simulink model "SR26"  (R2025a)
settings: Solver=FixedStepDiscrete  StartTime=0.0  StopTime=100  FixedStep=0.01  RelTol=1e-3  EnableMultiTasking=on
PreLoadFcn:
  | try, model_open; catch, disp('Error occurred while executing model pre-load callback: model_open.m'); disp('Please assure that the MATLAB working directory is set to the model directory before opening.'); end
InitFcn:
  | try, model_open; catch, end
values from neighbouring files (symbols this model uses):
  dt = 10.0    [SR26.sldd]
undefined symbols (not defined in the file or in its folder): BMSInputProcessing, GCM, raptor_get_safe_string, raptor_xcp_function, RegenEnable, StateCAN, Subsystem, TCEnable
libraries: Utilities x263, Raptor_lib x137, simulink x7, IO x5, APPS_BSPC x4, TorqueCommand x3, Cooling x3, StateMachine x2, DriveSpeed x2, ATCC x2, BrakePressure x2, ThrottlePosition x2
(part 2 of 4)

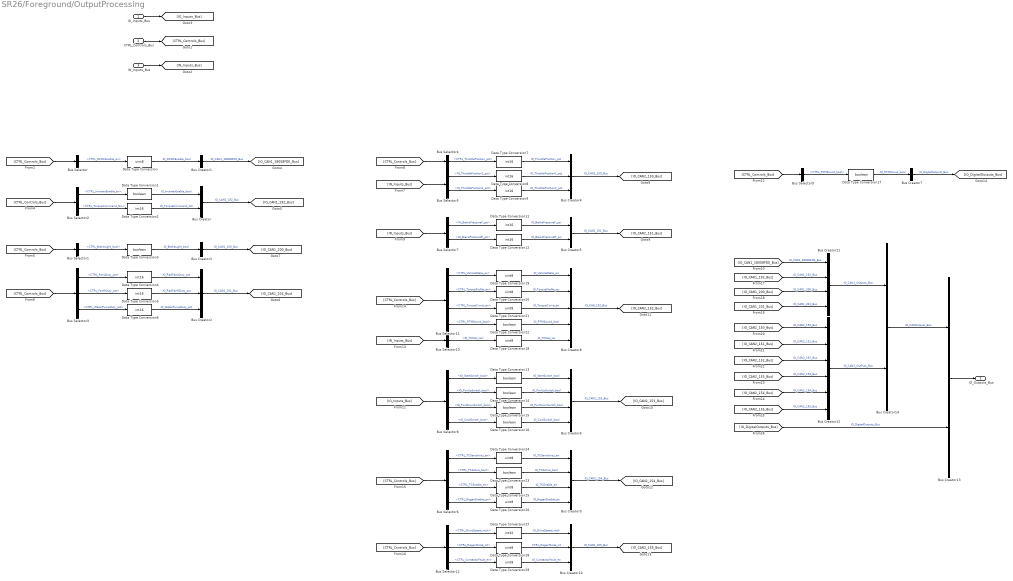
== system SR26/Foreground/OutputProcessing ==
  IO_Inputs_Bus : Inport
  CTRL_Controls_Bus : Inport  Port=2
  IN_Inputs_Bus : Inport  Port=3
  Bus Creator{,5,13..14} (4 alike) : BusCreator  Inputs=2
  Bus Creator1 : BusCreator  Inputs=1
  Bus Creator10 : BusCreator  Inputs=3
  Bus Creator11 : BusCreator  Inputs=4
  Bus Creator12 : BusCreator  Inputs=6
  Bus Creator2 : BusCreator  Inputs=3
  Bus Creator3 : BusCreator  Inputs=1
  Bus Creator4 : BusCreator  Inputs=3
  Bus Creator6 : BusCreator  Inputs=4
  Bus Creator7 : BusCreator  Inputs=1
  Bus Creator8 : BusCreator  Inputs=5
  Bus Creator9 : BusCreator  Inputs=4
  Bus Selector : BusSelector  OutputSignals=CTRL_DCDCEnable_en
  Bus Selector1 : BusSelector  OutputSignals=CTRL_BrakeLight_bool
  Bus Selector10 : BusSelector  OutputSignals=IN_TCDial_na
  Bus Selector11 : BusSelector  OutputSignals=CTRL_VehicleState_en,CTRL_TorqueProfile_en,CTRL_TorqueCurve_en,CTRL_RTMSound_bool
  Bus Selector12 : BusSelector  OutputSignals=CTRL_DriveSpeed_mph,CTRL_RegenMode_int,CTRL_ContactorFault_en
  Bus Selector2 : BusSelector  OutputSignals=CTRL_InverterEnable_en,CTRL_TorqueCommand_Nm
  Bus Selector3 : BusSelector  OutputSignals=CTRL_FanLDuty_pct,CTRL_FanRDuty_pct,CTRL_WaterPumpDuty_pct
  Bus Selector4 : BusSelector  OutputSignals=CTRL_ThrottlePosition_pct
  Bus Selector5 : BusSelector  OutputSignals=IN_ThrottlePosition_Bus.IN_ThrottlePosition1_pct,IN_ThrottlePosition_Bus.IN_ThrottlePosition2_pct
  Bus Selector6 : BusSelector  OutputSignals=CTRL_TCSensitivity_en,CTRL_TCActive_bool,CTRL_TCEnable_en,CTRL_RegenEnable_en
  Bus Selector7 : BusSelector  OutputSignals=IN_BrakePressure_Bus.IN_BrakePressureF_psi,IN_BrakePressure_Bus.IN_BrakePressureR_psi
  Bus Selector8 : BusSelector  OutputSignals=IO_DigitalInputs_Bus.IO_StartSwitch_bool,IO_DigitalInputs_Bus.IO_PwrUpSwitch_bool,IO_DigitalInputs_Bus.IO_PwrDownSwitch_bool,IO_DigitalInputs_Bus.IO_CoolSwitch_bool
  Bus Selector9 : BusSelector  OutputSignals=CTRL_RTMSound_bool
  Data Type Conversion{,18..21,24..26,28..29} (10 alike) : DataTypeConversion  OutDataTypeStr=uint8  SaturateOnIntegerOverflow=off  RndMeth=Floor
  Data Type Conversion{1,3,13..17,22..23} (9 alike) : DataTypeConversion  OutDataTypeStr=boolean  SaturateOnIntegerOverflow=off  RndMeth=Floor
  Data Type Conversion{2,4..9,11..12} (9 alike) : DataTypeConversion  OutDataTypeStr=int16  SaturateOnIntegerOverflow=off  RndMeth=Floor
  Data Type Conversion27 : DataTypeConversion  OutDataTypeStr=int32  SaturateOnIntegerOverflow=off  RndMeth=Floor
  IO_Outputs_Bus : Outport
  wires:
  IO_Inputs_Bus/1 -> [IO_Inputs_Bus]
  CTRL_Controls_Bus/1 -> [CTRL_Controls_Bus]
  IN_Inputs_Bus/1 -> [IN_Inputs_Bus]
  [CTRL_Controls_Bus] -> Bus Selector/1
  Bus Selector/1 -> Data Type Conversion/1  "<CTRL_DCDCEnable_en>"
  Bus Creator1/1 -> [IO_CAN1_18008FD0_Bus]  "IO_CAN1_18008FD0_Bus"
  [CTRL_Controls_Bus] -> Bus Selector2/1
  Bus Selector2/1 -> Data Type Conversion1/1  "<CTRL_InverterEnable_en>"
  Bus Selector2/2 -> Data Type Conversion2/1  "<CTRL_TorqueCommand_Nm>"
  Data Type Conversion2/1 -> Bus Creator/2  "IO_TorqueCommand_Nm"
  Data Type Conversion1/1 -> Bus Creator/1  "IO_InverterEnable_bool"
  Data Type Conversion/1 -> Bus Creator1/1  "IO_DCDCEnable_bool"
  Bus Creator/1 -> [IO_CAN1_192_Bus]  "IO_CAN1_192_Bus"
  [CTRL_Controls_Bus] -> Bus Selector1/1
  Bus Selector1/1 -> Data Type Conversion3/1  "<CTRL_BrakeLight_bool>"
  [CTRL_Controls_Bus] -> Bus Selector3/1
  Bus Selector3/1 -> Data Type Conversion4/1  "<CTRL_FanLDuty_pct>"
  Bus Selector3/2 -> Data Type Conversion5/1  "<CTRL_FanRDuty_pct>"
  Bus Selector3/3 -> Data Type Conversion6/1  "<CTRL_WaterPumpDuty_pct>"
  Data Type Conversion4/1 -> Bus Creator2/1  "IO_RadFanLDuty_pct"
  Data Type Conversion5/1 -> Bus Creator2/2  "IO_RadFanRDuty_pct"
  Data Type Conversion6/1 -> Bus Creator2/3  "IO_WaterPumpDuty_pct"
  Bus Creator2/1 -> [IO_CAN1_201_Bus]  "IO_CAN1_201_Bus"
  Data Type Conversion3/1 -> Bus Creator3/1  "IO_BrakeLight_bool"
  Bus Creator3/1 -> [IO_CAN1_200_Bus]  "IO_CAN1_200_Bus"
  [CTRL_Controls_Bus] -> Bus Selector4/1
  Bus Selector4/1 -> Data Type Conversion7/1  "<CTRL_ThrottlePosition_pct>"
  Data Type Conversion7/1 -> Bus Creator4/1  "IO_ThrottlePosition_pct"
  Bus Creator4/1 -> [IO_CAN2_150_Bus]  "IO_CAN1_150_Bus"
  [IN_Inputs_Bus] -> Bus Selector5/1
  Bus Selector5/1 -> Data Type Conversion8/1  "<IN_ThrottlePosition1_pct>"
  Bus Selector5/2 -> Data Type Conversion9/1  "<IN_ThrottlePosition2_pct>"
  Data Type Conversion8/1 -> Bus Creator4/2  "IO_ThrottlePosition1_pct"
  Data Type Conversion9/1 -> Bus Creator4/3  "IO_ThrottlePosition2_pct"
  Data Type Conversion12/1 -> Bus Creator5/2  "IO_BrakePressureR_psi"
  Data Type Conversion11/1 -> Bus Creator5/1  "IO_BrakePressureF_psi"
  [IN_Inputs_Bus] -> Bus Selector7/1
  Bus Creator5/1 -> [IO_CAN2_151_Bus]  "IO_CAN2_151_Bus"
  Bus Selector7/1 -> Data Type Conversion11/1  "<IN_BrakePressureF_psi>"
  Bus Selector7/2 -> Data Type Conversion12/1  "<IN_BrakePressureR_psi>"
  [IO_Inputs_Bus] -> Bus Selector8/1
  Bus Selector8/4 -> Data Type Conversion16/1  "<IO_CoolSwitch_bool>"
  Bus Selector8/3 -> Data Type Conversion15/1  "<IO_PwrDownSwitch_bool>"
  Bus Selector8/2 -> Data Type Conversion14/1  "<IO_PwrUpSwitch_bool>"
  Bus Selector8/1 -> Data Type Conversion13/1  "<IO_StartSwitch_bool>"
  Data Type Conversion13/1 -> Bus Creator6/1  "IO_StartSwitch_bool"
  Data Type Conversion14/1 -> Bus Creator6/2  "IO_PwrUpSwitch_bool"
  Data Type Conversion15/1 -> Bus Creator6/3  "IO_PwrDownSwitch_bool"
  Data Type Conversion16/1 -> Bus Creator6/4  "IO_CoolSwitch_bool"
  Bus Creator6/1 -> [IO_CAN2_153_Bus]  "IO_CAN2_153_Bus"
  [CTRL_Controls_Bus] -> Bus Selector9/1
  Bus Selector9/1 -> Data Type Conversion17/1  "<CTRL_RTMSound_bool>"
  Data Type Conversion17/1 -> Bus Creator7/1  "IO_RTMSound_bool"
  Bus Creator7/1 -> [IO_DigitalOutputs_Bus]  "IO_DigitalOutputs_Bus"
  Bus Creator8/1 -> [IO_CAN2_152_Bus]  "IO_CAN_152_Bus"
  Bus Selector10/1 -> Data Type Conversion18/1  "<IN_TCDial_na>"
  [IN_Inputs_Bus] -> Bus Selector10/1
  [CTRL_Controls_Bus] -> Bus Selector11/1
  Bus Selector11/1 -> Data Type Conversion19/1  "<CTRL_VehicleState_en>"
  Bus Selector11/2 -> Data Type Conversion20/1  "<CTRL_TorqueProfile_en>"
  Bus Selector11/3 -> Data Type Conversion21/1  "<CTRL_TorqueCurve_en>"
  Bus Selector11/4 -> Data Type Conversion22/1  "<CTRL_RTMSound_bool>"
  Data Type Conversion19/1 -> Bus Creator8/1  "IO_VehicleState_en"
  Data Type Conversion20/1 -> Bus Creator8/2  "IO_TorqueProfile_en"
  Data Type Conversion21/1 -> Bus Creator8/3  "IO_TorqueCurve_en"
  Data Type Conversion22/1 -> Bus Creator8/4  "IO_RTMSound_bool"
  Data Type Conversion18/1 -> Bus Creator8/5  "IO_TCDial_na"
  [CTRL_Controls_Bus] -> Bus Selector6/1
  Bus Selector6/1 -> Data Type Conversion24/1  "<CTRL_TCSensitivity_en>"
  Bus Selector6/2 -> Data Type Conversion23/1  "<CTRL_TCActive_bool>"
  Bus Selector6/3 -> Data Type Conversion25/1  "<CTRL_TCEnable_en>"
  Bus Selector6/4 -> Data Type Conversion26/1  "<CTRL_RegenEnable_en>"
  Data Type Conversion23/1 -> Bus Creator9/2  "IO_TCActive_bool"
  Data Type Conversion24/1 -> Bus Creator9/1  "IO_TCSensitivity_en"
  Data Type Conversion25/1 -> Bus Creator9/3  "IO_TCEnable_en"
  Data Type Conversion26/1 -> Bus Creator9/4  "IO_RegenEnable_en"
  Bus Creator9/1 -> [IO_CAN2_154_Bus]  "IO_CAN2_154_Bus"
  [CTRL_Controls_Bus] -> Bus Selector12/1
  Bus Selector12/1 -> Data Type Conversion27/1  "<CTRL_DriveSpeed_mph>"
  Bus Selector12/2 -> Data Type Conversion28/1  "<CTRL_RegenMode_int>"
  Bus Selector12/3 -> Data Type Conversion29/1  "<CTRL_ContactorFault_en>"
  Data Type Conversion29/1 -> Bus Creator10/3  "IO_ContactorFault_en"
  Data Type Conversion28/1 -> Bus Creator10/2  "CTRL_RegenMode_int"
  Data Type Conversion27/1 -> Bus Creator10/1  "IO_DriveSpeed_mph"
  Bus Creator10/1 -> [IO_CAN2_155_Bus]  "IO_CAN2_155_Bus"
  [IO_CAN1_18008FD0_Bus] -> Bus Creator11/1  "IO_CAN1_18008FD0_Bus"
  [IO_CAN1_192_Bus] -> Bus Creator11/2  "IO_CAN1_192_Bus"
  [IO_CAN1_200_Bus] -> Bus Creator11/3  "IO_CAN1_200_Bus"
  [IO_CAN1_201_Bus] -> Bus Creator11/4  "IO_CAN1_201_Bus"
  [IO_CAN2_150_Bus] -> Bus Creator12/1  "IO_CAN2_150_Bus"
  [IO_CAN2_151_Bus] -> Bus Creator12/2  "IO_CAN2_151_Bus"
  [IO_CAN2_152_Bus] -> Bus Creator12/3  "IO_CAN2_152_Bus"
  [IO_CAN2_153_Bus] -> Bus Creator12/4  "IO_CAN2_153_Bus"
  [IO_CAN2_154_Bus] -> Bus Creator12/5  "IO_CAN2_154_Bus"
  [IO_CAN2_155_Bus] -> Bus Creator12/6  "IO_CAN2_155_Bus"
  [IO_DigitalOutputs_Bus] -> Bus Creator13/2  "IO_DigitalOutputs_Bus"
  Bus Creator13/1 -> IO_Outputs_Bus/1
  Bus Creator11/1 -> Bus Creator14/1  "IO_CAN1_Outputs_Bus"
  Bus Creator12/1 -> Bus Creator14/2  "IO_CAN2_OutPuts_Bus"
  Bus Creator14/1 -> Bus Creator13/1  "IO_CANOutputs_Bus"

== system SR26/Power Up_Down/Background ==
  note: Notes :
      | - Calling the shutdown task stops the foreground tasks. However, background tasks continue, so the reading of key switch must be in this subsystem to allow the module
      | to resume operation (by calling the startup task) if keyswitch is turned back on before the module actually turns off.
      | - The Startup Event is automatically called when the module is powered on after being completely off. The FgndTasksStopped data store prevents the Startup Event from being called twice in this scenario.
  f : TriggerPort  TriggerType=function-call  VariantControl=Variant  ZeroCross=off
  Debounce : Subsystem
  Logical Operator1 : Logic  Operator=OR  OutDataTypeStr=boolean
  Logical Operator2 : Logic  Operator=OR  Inputs=3  OutDataTypeStr=boolean
  Raise Shutdown Event : Subsystem  TreatAsAtomicUnit=on
  Raise Startup Event : Subsystem  TreatAsAtomicUnit=on
  Store EEPROM : Subsystem  TreatAsAtomicUnit=on
  Unit Delay : UnitDelay  SampleTime=-1  HasFrameUpgradeWarning=on
  Unit Delay1 : UnitDelay  SampleTime=-1  HasFrameUpgradeWarning=on
  raptor_data_def : Raptor_lib/Data Storage/raptor_data_def  dataName='KeySw_Bgnd'  initValue=0  dataType=boolean  storage=Volatile (RAM)  calVisible=on  calType=Measurement  calDispType=Number  calEnum={'False', 'True'}  calGain=1.0  calOffset=0  calMin=-Inf  calMax=Inf  calFormat='-1'  calUnit='Bool'  calHelp='Key switch reading from background task'  calAccess=1  calFunction=group  calDispHeaders=off  calColHeaders={'Col1' 'Col2' 'Col3'}  calRowHeaders={'Row1' 'Row2' 'Row3'}
      settings: SourceProductName=Raptor
  raptor_data_def1 : Raptor_lib/Data Storage/raptor_data_def  dataName='KeepModuleOn'  initValue=0  dataType=boolean  storage=Volatile (RAM)  calVisible=on  calType=Measurement  calDispType=Number  calEnum={'False', 'True'}  calGain=1.0  calOffset=0  calMin=-Inf  calMax=Inf  calFormat='-1'  calUnit='Bool'  calHelp='Boolean indicating module to be kept on'  calAccess=1  calFunction=group  calDispHeaders=off  calColHeaders={'Col1' 'Col2' 'Col3'}  calRowHeaders={'Row1' 'Row2' 'Row3'}
      settings: SourceProductName=Raptor
  raptor_data_read : Raptor_lib/Data Storage/raptor_data_read  dataName='FgndTasksStopped'  dataShape=Scalar  idxSource=Input  idxRow=1  idxCol=1
      settings: SourceProductName=Raptor
  raptor_data_read1 : Raptor_lib/Data Storage/raptor_data_read  dataName='KeepModuleOn'  dataShape=Scalar  idxSource=Input  idxRow=1  idxCol=1
      settings: SourceProductName=Raptor
  raptor_data_write : Raptor_lib/Data Storage/raptor_data_write  dataName='KeySw_Bgnd'  dataShape=Scalar  idxSource=Input Port  idxRow=1  idxCol=1
      settings: SourceProductName=Raptor
  raptor_digital_in : Raptor_lib/Input & Output/raptor_digital_in  resourceValues=WAKE_INPUT1|INPUT33|INPUT34|INPUT35|INPUT36|INPUT37|INPUT38|INPUT39|INPUT40|(None)  resource=WAKE_INPUT1  pullUDValues=2.9k PD  pullUD=2.9k PD  upperThres=1.980  lowerThres=1.320
      settings: SourceProductName=Raptor
  raptor_digital_out : Raptor_lib/Input & Output/raptor_digital_out  resourceValues=OUTPUT9|OUTPUT21|OUTPUT22|OUTPUT23|OUTPUT24|(None)|OUTPUT1|OUTPUT2|OUTPUT3|OUTPUT4|OUTPUT5|OUTPUT6|OUTPUT7|OUTPUT8|OUTPUT10|OUTPUT11|OUTPUT25|OUTPUT26|OUTPUT27|OUTPUT28|OUTPUT29|OUTPUT30|OUTPUT31|OUTPUT32|OUTPUT33|OUTPUT34|OUTPUT35|OUTPUT36|OUTPUT37|OUTPUT38|OUTPUT39|OUTPUT40|OUTPUT41|OUTPUT42|OUTPUT43|OUTPUT44|OUTPUT45|OUTPUT46|OUTPUT47|OUTPUT48|POWER_HOLD  resource=POWER_HOLD  driverTypeValues=(None)  driverType=(None)
      settings: SourceProductName=Raptor
  raptor_sfun_nv_status : Raptor_lib/Data Storage/raptor_sfun_nv_status  showStatus=Store In Progess
      settings: SourceProductName=Raptor
  wires:
  raptor_data_read/1 -> Raise Startup Event/Enable
  raptor_digital_in/1 -> Debounce/1(In)
  Logical Operator2/1 -> raptor_digital_out/1
  Unit Delay/1 -> Store EEPROM/Trigger, Unit Delay1/1
  Logical Operator1/1 -> Logical Operator2/2, Raise Startup Event/Trigger, Raise Shutdown Event/Trigger, Unit Delay/1
  Unit Delay1/1 -> Logical Operator2/3
  raptor_sfun_nv_status/1 -> Logical Operator2/1
  raptor_data_read1/1 -> Logical Operator1/2
  Debounce/1(Out) -> raptor_data_write/1, Logical Operator1/1

== system SR26/Foreground/Controls Algorithm/APPS_BSPC ==
  IN_Inputs_Bus : Inport
  function : TriggerPort  TriggerType=function-call  VariantControl=(inherit)
  APPS : APPS_BSPC/APPS  SystemSampleTime=-1  VariantActivationTime=update diagram  EmptyChoice=off  PassThrough=off  PassThroughVariantControl=(default)  EmptyChoiceVariantControl=(default)  AllowFlexibleInterface=on  Latency=0  AutoFrameSizeCalculation=off
  BSPC : APPS_BSPC/BSPC  SystemSampleTime=-1  VariantActivationTime=update diagram  EmptyChoice=off  PassThrough=off  PassThroughVariantControl=(default)  EmptyChoiceVariantControl=(default)  AllowFlexibleInterface=on  Latency=0  AutoFrameSizeCalculation=off
  BSPCReset : APPS_BSPC/BSPCReset  SystemSampleTime=-1  VariantActivationTime=update diagram  EmptyChoice=off  PassThrough=off  PassThroughVariantControl=(default)  EmptyChoiceVariantControl=(default)  AllowFlexibleInterface=on  Latency=0  AutoFrameSizeCalculation=off
  Bus Selector : BusSelector  OutputSignals=IN_ThrottlePosition_Bus.IN_ThrottlePosition1_pct,IN_ThrottlePosition_Bus.IN_ThrottlePosition2_pct,IN_BrakePressure_Bus.IN_BrakePressureF_psi,IN_BrakePressure_Bus.IN_BrakePressureR_psi
  ThrottleSignal : APPS_BSPC/ThrottleSignal  SystemSampleTime=-1  VariantActivationTime=update diagram  EmptyChoice=off  PassThrough=off  PassThroughVariantControl=(default)  EmptyChoiceVariantControl=(default)  AllowFlexibleInterface=on  Latency=0  AutoFrameSizeCalculation=off
  CTRL_ThrottlePosition_pct : Outport
  wires:
  IN_Inputs_Bus/1 -> Bus Selector/1
  ThrottleSignal/1 -> CTRL_ThrottlePosition_pct/1
  Bus Selector/1 -> BSPC/1, BSPCReset/1, ThrottleSignal/1, APPS/1  "<IN_ThrottlePosition1_pct>"
  Bus Selector/2 -> BSPC/2, BSPCReset/2, ThrottleSignal/2, APPS/2  "<IN_ThrottlePosition2_pct>"
  Bus Selector/3 -> BSPC/3  "<IN_BrakePressureF_psi>"
  Bus Selector/4 -> BSPC/4  "<IN_BrakePressureR_psi>"

== system SR26/Foreground/Controls Algorithm/BrakeLight ==
  IN_Inputs_Bus : Inport
  function : TriggerPort  TriggerType=function-call  VariantControl=(inherit)
  BrakeLight : Brakes/BrakeLight  SystemSampleTime=-1  VariantActivationTime=update diagram  EmptyChoice=off  PassThrough=off  PassThroughVariantControl=(default)  EmptyChoiceVariantControl=(default)  AllowFlexibleInterface=on  Latency=0  AutoFrameSizeCalculation=off
  Bus Selector : BusSelector  OutputSignals=IN_BrakePressure_Bus.IN_BrakePressureF_psi,IN_BrakePressure_Bus.IN_BrakePressureR_psi
  CTRL_BrakeLight_bool : Outport
  wires:
  IN_Inputs_Bus/1 -> Bus Selector/1
  Bus Selector/1 -> BrakeLight/1  "<IN_BrakePressureF_psi>"
  Bus Selector/2 -> BrakeLight/2  "<IN_BrakePressureR_psi>"
  BrakeLight/1 -> CTRL_BrakeLight_bool/1

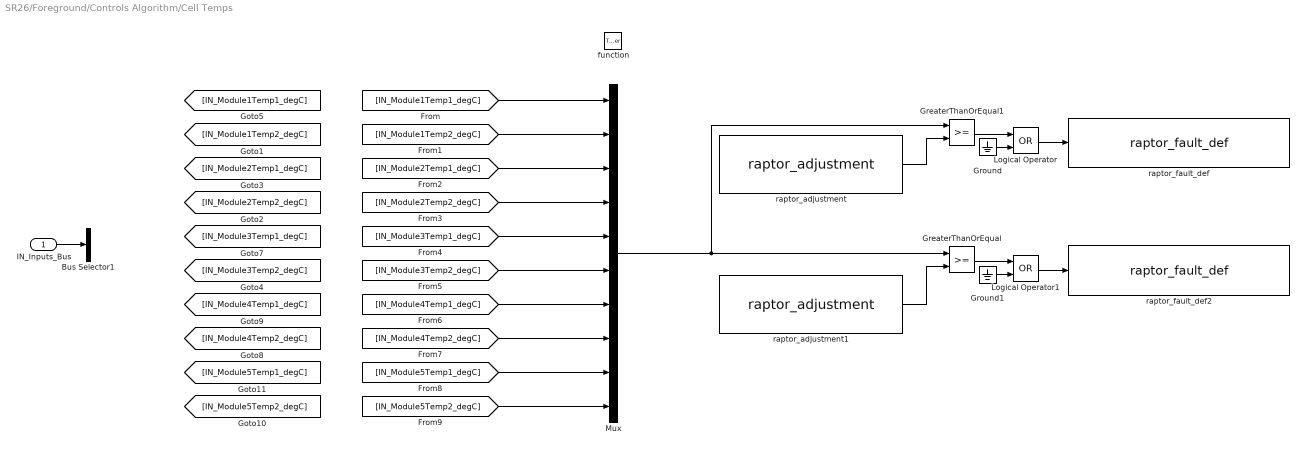
== system SR26/Foreground/Controls Algorithm/Cell Temps ==
  IN_Inputs_Bus : Inport
  function : TriggerPort  TriggerType=function-call  VariantControl=(inherit)
  Bus Selector1 : BusSelector  OutputSignals=IO_DigitalInputs_Bus.IO_CoolSwitch_bool
  GreaterThanOrEqual : RelationalOperator  OutDataTypeStr=boolean  RndMeth=Simplest  InputSameDT=off
  GreaterThanOrEqual1 : RelationalOperator  OutDataTypeStr=boolean  RndMeth=Simplest  InputSameDT=off
  Ground : Ground
  Ground1 : Ground
  Logical Operator : Logic  Operator=OR  AllPortsSameDT=off  OutDataTypeStr=boolean
  Logical Operator1 : Logic  Operator=OR  AllPortsSameDT=off  OutDataTypeStr=boolean
  Mux : Mux  Inputs=10
  raptor_adjustment : Raptor_lib/Data Storage/raptor_adjustment  paramName='CTRL_ModuleUnderThresh_degC'  nameSource=Parameter  initValue=-10  dataType=double  storage=Calibration  calDispType=Number  calEnum={'False', 'True'}  calGain=1.0  calOffset=0.0  calMax=inf  calMin=-inf  calFormat='-1'  calUnit=''  calHelp=''  calAccess=1  calFunction=raptor_xcp_function(gcb)  calDispHeaders=off  calColHeaders={'Col1' 'Col2' 'Col3'}  calRowHeaders={'Row1' 'Row2' 'Row3'}
      settings: SourceProductName=Raptor
  raptor_adjustment1 : Raptor_lib/Data Storage/raptor_adjustment  paramName='CTRL_ModuleOverTempThresh_degC'  nameSource=Parameter  initValue=55  dataType=double  storage=Calibration  calDispType=Number  calEnum={'False', 'True'}  calGain=1.0  calOffset=0.0  calMax=inf  calMin=-inf  calFormat='-1'  calUnit=''  calHelp=''  calAccess=1  calFunction=raptor_xcp_function(gcb)  calDispHeaders=off  calColHeaders={'Col1' 'Col2' 'Col3'}  calRowHeaders={'Row1' 'Row2' 'Row3'}
      settings: SourceProductName=Raptor
  raptor_fault_def : Raptor_lib/Faults/raptor_fault_def  faultName='CTRL_ModuleUnderTempFault'  persist=off  sticky=off  emisRelated=off  permanent=off  singleTrip=off  clearMethod=Standard  xLimit=25  yLimit=50  calEnable=on  addDisable=off  calAccess=1  calFunction='System | FaultManager'
      settings: SourceProductName=Raptor
  raptor_fault_def2 : Raptor_lib/Faults/raptor_fault_def  faultName='CTRL_ModuleOverTempTempFault'  persist=off  sticky=off  emisRelated=off  permanent=off  singleTrip=off  clearMethod=Standard  xLimit=25  yLimit=50  calEnable=on  addDisable=off  calAccess=1  calFunction='System | FaultManager'
      settings: SourceProductName=Raptor
  wires:
  IN_Inputs_Bus/1 -> Bus Selector1/1
  [IN_Module1Temp1_degC] -> Mux/1
  [IN_Module1Temp2_degC] -> Mux/2
  [IN_Module2Temp1_degC] -> Mux/3
  [IN_Module2Temp2_degC] -> Mux/4
  [IN_Module3Temp1_degC] -> Mux/5
  [IN_Module3Temp2_degC] -> Mux/6
  [IN_Module4Temp1_degC] -> Mux/7
  [IN_Module4Temp2_degC] -> Mux/8
  [IN_Module5Temp1_degC] -> Mux/9
  [IN_Module5Temp2_degC] -> Mux/10
  Mux/1 -> GreaterThanOrEqual1/1, GreaterThanOrEqual/1
  raptor_adjustment/1 -> GreaterThanOrEqual1/2
  raptor_adjustment1/1 -> GreaterThanOrEqual/2
  GreaterThanOrEqual1/1 -> Logical Operator/1
  Ground/1 -> Logical Operator/2
  Ground1/1 -> Logical Operator1/2
  GreaterThanOrEqual/1 -> Logical Operator1/1
  Logical Operator/1 -> raptor_fault_def/1
  Logical Operator1/1 -> raptor_fault_def2/1

== system SR26/Foreground/Controls Algorithm/ClearAllFaults ==
  function : TriggerPort  TriggerType=function-call  VariantControl=(inherit)
  raptor_fault_clear : Raptor_lib/Faults/raptor_fault_clear  faultSource=All  faultName='myFault'
      settings: SourceProductName=Raptor

== system SR26/Foreground/Controls Algorithm/RTMSound ==
  CTRL_VehicleState_en : Inport
  function : TriggerPort  TriggerType=function-call  VariantControl=(inherit)
  RTMSound : StateMachine/RTMSound  SystemSampleTime=-1  VariantActivationTime=update diagram  EmptyChoice=off  PassThrough=off  PassThroughVariantControl=(default)  EmptyChoiceVariantControl=(default)  AllowFlexibleInterface=on  Latency=0  AutoFrameSizeCalculation=off
  CTRL_RTMSound_bool : Outport
  wires:
  RTMSound/1 -> CTRL_RTMSound_bool/1
  CTRL_VehicleState_en/1 -> RTMSound/1

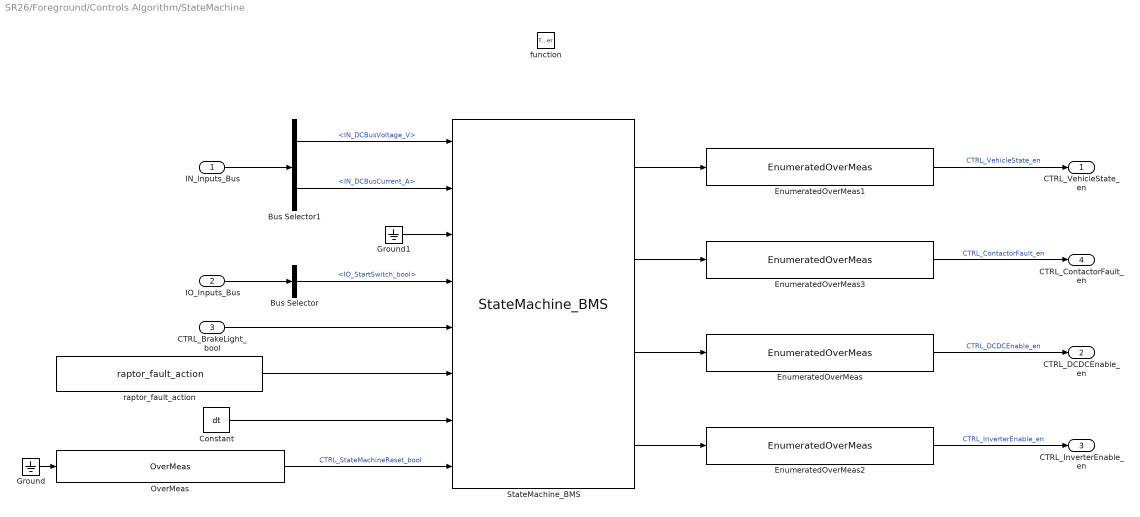
== system SR26/Foreground/Controls Algorithm/StateMachine ==
  IN_Inputs_Bus : Inport
  IO_Inputs_Bus : Inport  Port=2
  CTRL_BrakeLight_bool : Inport  Port=3
  function : TriggerPort  TriggerType=function-call  VariantControl=(inherit)
  Bus Selector : BusSelector  OutputSignals=IO_DigitalInputs_Bus.IO_StartSwitch_bool
  Bus Selector1 : BusSelector  OutputSignals=IN_CAN1_PM100DX_Bus.IN_DCBusVoltage_V,IN_CAN1_PM100DX_Bus.IN_DCBusCurrent_A
  Constant : Constant  Value=dt  OutDataTypeStr=uint32
  EnumeratedOverMeas : Utilities/EnumeratedOverMeas  sigName='CTRL_DCDCEnable_en'  enumName='DCDCEnable'
  EnumeratedOverMeas1 : Utilities/EnumeratedOverMeas  sigName='CTRL_VehicleState_en'  enumName='VehicleState'
  EnumeratedOverMeas2 : Utilities/EnumeratedOverMeas  sigName='CTRL_InverterEnable_en'  enumName='InverterEnable'
  EnumeratedOverMeas3 : Utilities/EnumeratedOverMeas  sigName='CTRL_ContactorFault_en'  enumName='ContactorFault'
  Ground : Ground
  Ground1 : Ground
  OverMeas : Utilities/OverMeas  sigName='CTRL_StateMachineReset_bool'  minimum=0  maximum=1
  StateMachine_BMS : StateMachine/StateMachine_BMS  SystemSampleTime=-1  VariantActivationTime=update diagram  EmptyChoice=off  PassThrough=off  PassThroughVariantControl=(default)  EmptyChoiceVariantControl=(default)  AllowFlexibleInterface=on  Latency=0  AutoFrameSizeCalculation=off
  raptor_fault_action : Raptor_lib/Faults/raptor_fault_action  actionName='myFaultAction'  calVisible=off  calAccess=1  calFunction='System | FaultManager | FaultAction'
      settings: SourceProductName=Raptor
  CTRL_VehicleState_en : Outport
  CTRL_DCDCEnable_en : Outport  Port=2
  CTRL_InverterEnable_en : Outport  Port=3
  CTRL_ContactorFault_en : Outport  Port=4
  wires:
  IO_Inputs_Bus/1 -> Bus Selector/1
  Bus Selector/1 -> StateMachine_BMS/4  "<IO_StartSwitch_bool>"
  IN_Inputs_Bus/1 -> Bus Selector1/1
  Bus Selector1/1 -> StateMachine_BMS/1  "<IN_DCBusVoltage_V>"
  Ground/1 -> OverMeas/1
  CTRL_BrakeLight_bool/1 -> StateMachine_BMS/5
  raptor_fault_action/1 -> StateMachine_BMS/6
  Constant/1 -> StateMachine_BMS/7
  OverMeas/1 -> StateMachine_BMS/8  "CTRL_StateMachineReset_bool"
  StateMachine_BMS/3 -> EnumeratedOverMeas/1
  StateMachine_BMS/1 -> EnumeratedOverMeas1/1
  StateMachine_BMS/4 -> EnumeratedOverMeas2/1
  EnumeratedOverMeas/1 -> CTRL_DCDCEnable_en/1  "CTRL_DCDCEnable_en"
  EnumeratedOverMeas2/1 -> CTRL_InverterEnable_en/1  "CTRL_InverterEnable_en"
  EnumeratedOverMeas1/1 -> CTRL_VehicleState_en/1  "CTRL_VehicleState_en"
  StateMachine_BMS/2 -> EnumeratedOverMeas3/1
  EnumeratedOverMeas3/1 -> CTRL_ContactorFault_en/1  "CTRL_ContactorFault_en"
  Ground1/1 -> StateMachine_BMS/3
  Bus Selector1/2 -> StateMachine_BMS/2  "<IN_DCBusCurrent_A>"

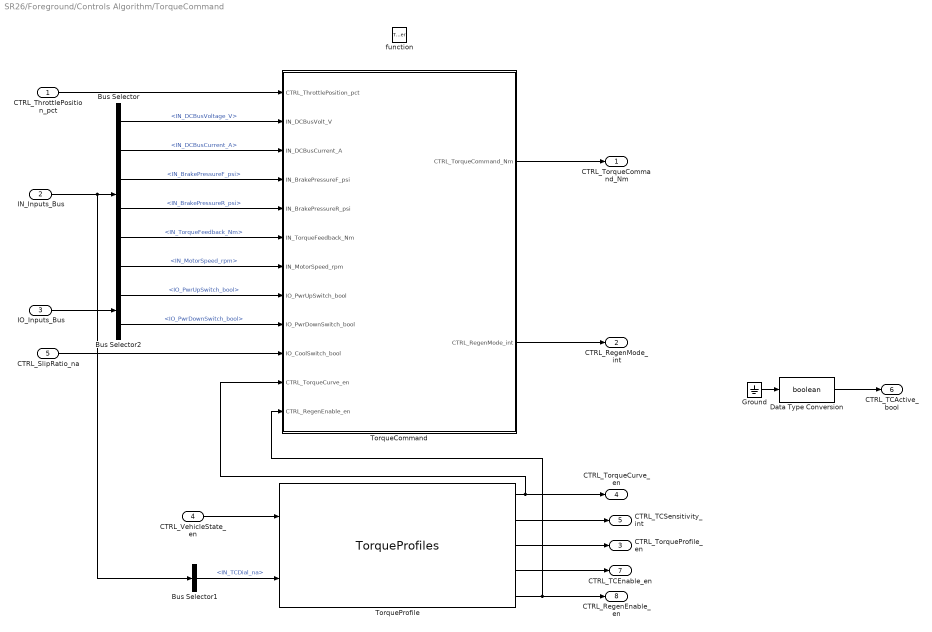
== system SR26/Foreground/Controls Algorithm/TorqueCommand ==
  CTRL_ThrottlePosition_pct : Inport
  IN_Inputs_Bus : Inport  Port=2
  IO_Inputs_Bus : Inport  Port=3
  CTRL_VehicleState_en : Inport  Port=4
  CTRL_SlipRatio_na : Inport  Port=5
  function : TriggerPort  TriggerType=function-call  VariantControl=(inherit)
  Bus Selector : BusSelector  OutputSignals=IN_CAN1_PM100DX_Bus.IN_DCBusVoltage_V,IN_CAN1_PM100DX_Bus.IN_DCBusCurrent_A,IN_BrakePressure_Bus.IN_BrakePressureF_psi,IN_BrakePressure_Bus.IN_BrakePressureR_psi,IN_CAN1_PM100DX_Bus.IN_TorqueFeedback_Nm,IN_CAN1_PM100DX_Bus.IN_MotorSpeed_rpm
  Bus Selector1 : BusSelector  OutputSignals=IN_TCDial_na
  Bus Selector2 : BusSelector  OutputSignals=IO_DigitalInputs_Bus.IO_PwrUpSwitch_bool,IO_DigitalInputs_Bus.IO_PwrDownSwitch_bool
  Data Type Conversion : DataTypeConversion  OutDataTypeStr=boolean  SaturateOnIntegerOverflow=off  RndMeth=Floor
  Ground : Ground
  TorqueCommand : Subsystem  AncestorBlock=TorqueCommand/TorqueCommand
  TorqueProfile : TorqueCommand/TorqueProfiles  SystemSampleTime=-1  VariantActivationTime=update diagram  EmptyChoice=off  PassThrough=off  PassThroughVariantControl=(default)  EmptyChoiceVariantControl=(default)  AllowFlexibleInterface=on  Latency=0  AutoFrameSizeCalculation=off
  CTRL_TorqueCommand_Nm : Outport  VectorParamsAs1DForOutWhenUnconnected=off
  CTRL_RegenMode_int : Outport  Port=2  VectorParamsAs1DForOutWhenUnconnected=off
  CTRL_TorqueProfile_en : Outport  Port=3  VectorParamsAs1DForOutWhenUnconnected=off
  CTRL_TorqueCurve_en : Outport  Port=4  VectorParamsAs1DForOutWhenUnconnected=off
  CTRL_TCSensitivity_int : Outport  Port=5  VectorParamsAs1DForOutWhenUnconnected=off
  CTRL_TCActive_bool : Outport  Port=6  VectorParamsAs1DForOutWhenUnconnected=off
  CTRL_TCEnable_en : Outport  Port=7  VectorParamsAs1DForOutWhenUnconnected=off
  CTRL_RegenEnable_en : Outport  Port=8  VectorParamsAs1DForOutWhenUnconnected=off
  wires:
  CTRL_ThrottlePosition_pct/1 -> TorqueCommand/1(CTRL_ThrottlePosition_pct)
  TorqueCommand/1(CTRL_TorqueCommand_Nm) -> CTRL_TorqueCommand_Nm/1
  IN_Inputs_Bus/1 -> Bus Selector1/1, Bus Selector/1
  TorqueProfile/1 -> TorqueCommand/11(CTRL_TorqueCurve_en), CTRL_TorqueCurve_en/1
  IO_Inputs_Bus/1 -> Bus Selector2/1
  Bus Selector1/1 -> TorqueProfile/2  "<IN_TCDial_na>"
  TorqueProfile/2 -> CTRL_TCSensitivity_int/1
  TorqueProfile/3 -> CTRL_TorqueProfile_en/1
  CTRL_VehicleState_en/1 -> TorqueProfile/1
  Bus Selector2/1 -> TorqueCommand/8(IO_PwrUpSwitch_bool)  "<IO_PwrUpSwitch_bool>"
  Bus Selector2/2 -> TorqueCommand/9(IO_PwrDownSwitch_bool)  "<IO_PwrDownSwitch_bool>"
  Bus Selector/3 -> TorqueCommand/4(IN_BrakePressureF_psi)  "<IN_BrakePressureF_psi>"
  Bus Selector/4 -> TorqueCommand/5(IN_BrakePressureR_psi)  "<IN_BrakePressureR_psi>"
  Bus Selector/5 -> TorqueCommand/6(IN_TorqueFeedback_Nm)  "<IN_TorqueFeedback_Nm>"
  Bus Selector/1 -> TorqueCommand/2(IN_DCBusVolt_V)  "<IN_DCBusVoltage_V>"
  Bus Selector/2 -> TorqueCommand/3(IN_DCBusCurrent_A)  "<IN_DCBusCurrent_A>"
  TorqueProfile/4 -> CTRL_TCEnable_en/1
  TorqueProfile/5 -> TorqueCommand/12(CTRL_RegenEnable_en), CTRL_RegenEnable_en/1
  Ground/1 -> Data Type Conversion/1
  Data Type Conversion/1 -> CTRL_TCActive_bool/1
  CTRL_SlipRatio_na/1 -> TorqueCommand/10(IO_CoolSwitch_bool)
  TorqueCommand/2(CTRL_RegenMode_int) -> CTRL_RegenMode_int/1
  Bus Selector/6 -> TorqueCommand/7(IN_MotorSpeed_rpm)  "<IN_MotorSpeed_rpm>"

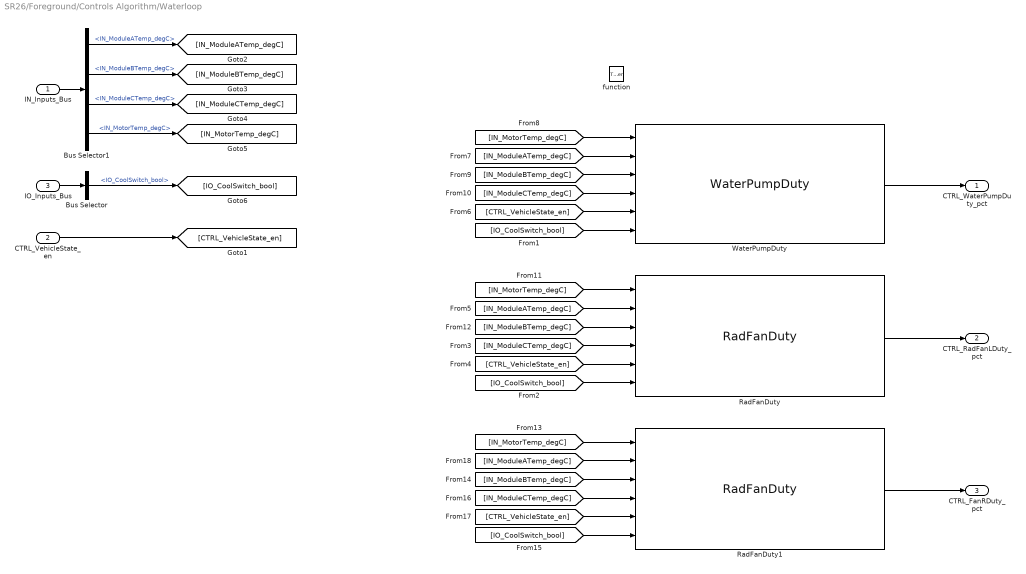
== system SR26/Foreground/Controls Algorithm/Waterloop ==
  IN_Inputs_Bus : Inport
  CTRL_VehicleState_en : Inport  Port=2
  IO_Inputs_Bus : Inport  Port=3
  function : TriggerPort  TriggerType=function-call  VariantControl=(inherit)
  Bus Selector : BusSelector  OutputSignals=IO_DigitalInputs_Bus.IO_CoolSwitch_bool
  Bus Selector1 : BusSelector  OutputSignals=IN_CAN1_PM100DX_Bus.IN_ModuleATemp_degC,IN_CAN1_PM100DX_Bus.IN_ModuleBTemp_degC,IN_CAN1_PM100DX_Bus.IN_ModuleCTemp_degC,IN_CAN1_PM100DX_Bus.IN_MotorTemp_degC
  RadFanDuty : Cooling/RadFanDuty  pos='L'
  RadFanDuty1 : Cooling/RadFanDuty  pos='R'
  WaterPumpDuty : Cooling/WaterPumpDuty
  CTRL_WaterPumpDuty_pct : Outport
  CTRL_RadFanLDuty_pct : Outport  Port=2
  CTRL_FanRDuty_pct : Outport  Port=3
  wires:
  RadFanDuty/1 -> CTRL_RadFanLDuty_pct/1
  WaterPumpDuty/1 -> CTRL_WaterPumpDuty_pct/1
  IO_Inputs_Bus/1 -> Bus Selector/1
  Bus Selector/1 -> [IO_CoolSwitch_bool]  "<IO_CoolSwitch_bool>"
  CTRL_VehicleState_en/1 -> [CTRL_VehicleState_en]
  [CTRL_VehicleState_en] -> WaterPumpDuty/5
  [IO_CoolSwitch_bool] -> WaterPumpDuty/6
  RadFanDuty1/1 -> CTRL_FanRDuty_pct/1
  IN_Inputs_Bus/1 -> Bus Selector1/1
  [IN_ModuleATemp_degC] -> WaterPumpDuty/2
  [IN_MotorTemp_degC] -> WaterPumpDuty/1
  [IN_ModuleBTemp_degC] -> WaterPumpDuty/3
  [IN_ModuleCTemp_degC] -> WaterPumpDuty/4
  [IN_ModuleCTemp_degC] -> RadFanDuty/4
  [IN_ModuleBTemp_degC] -> RadFanDuty/3
  [IN_MotorTemp_degC] -> RadFanDuty/1
  [IN_ModuleATemp_degC] -> RadFanDuty/2
  [IO_CoolSwitch_bool] -> RadFanDuty/6
  [CTRL_VehicleState_en] -> RadFanDuty/5
  [CTRL_VehicleState_en] -> RadFanDuty1/5
  [IO_CoolSwitch_bool] -> RadFanDuty1/6
  [IN_ModuleATemp_degC] -> RadFanDuty1/2
  [IN_MotorTemp_degC] -> RadFanDuty1/1
  [IN_ModuleBTemp_degC] -> RadFanDuty1/3
  [IN_ModuleCTemp_degC] -> RadFanDuty1/4
  Bus Selector1/1 -> [IN_ModuleATemp_degC]  "<IN_ModuleATemp_degC>"
  Bus Selector1/2 -> [IN_ModuleBTemp_degC]  "<IN_ModuleBTemp_degC>"
  Bus Selector1/3 -> [IN_ModuleCTemp_degC]  "<IN_ModuleCTemp_degC>"
  Bus Selector1/4 -> [IN_MotorTemp_degC]  "<IN_MotorTemp_degC>"

== system SR26/Foreground/Controls Algorithm/Wheels ==
  IN_Inputs_Bus : Inport
  function : TriggerPort  TriggerType=function-call  VariantControl=(inherit)
  Add : Sum
  Add1 : Sum
  Bus Selector : BusSelector  OutputSignals=IN_CAN1_ATCCF_Bus.IN_WheelSpeedFL_rpm,IN_CAN1_ATCCF_Bus.IN_WheelSpeedFR_rpm,IN_CAN1_ATCCR_Bus.IN_WheelSpeedRL_rpm,IN_CAN1_ATCCR_Bus.IN_WheelSpeedRR_rpm
  Constant : Constant  Value=2
  Constant1 : Constant  Value=2
  Divide : Product  Inputs=*/
  Divide1 : Product  Inputs=*/
  DriveSpeed : DriveSpeed/DriveSpeed  SystemSampleTime=-1  VariantActivationTime=update diagram  EmptyChoice=off  PassThrough=off  PassThroughVariantControl=(default)  EmptyChoiceVariantControl=(default)  AllowFlexibleInterface=on  Latency=0  AutoFrameSizeCalculation=off
  SlipRatio : DriveSpeed/SlipRatio  SystemSampleTime=-1  VariantActivationTime=update diagram  EmptyChoice=off  PassThrough=off  PassThroughVariantControl=(default)  EmptyChoiceVariantControl=(default)  AllowFlexibleInterface=on  Latency=0  AutoFrameSizeCalculation=off
  CTRL_DriveSpeed_mph : Outport
  CTRL_SlipRatio_na : Outport  Port=2
  wires:
  IN_Inputs_Bus/1 -> Bus Selector/1
  DriveSpeed/1 -> CTRL_DriveSpeed_mph/1
  Bus Selector/1 -> Add/1  "<IN_WheelSpeedFL_rpm>"
  Bus Selector/2 -> Add/2  "<IN_WheelSpeedFR_rpm>"
  Add/1 -> Divide/1
  Constant/1 -> Divide/2
  Constant1/1 -> Divide1/2
  Add1/1 -> Divide1/1
  Bus Selector/4 -> Add1/2  "<IN_WheelSpeedRR_rpm>"
  Bus Selector/3 -> Add1/1  "<IN_WheelSpeedRL_rpm>"
  Divide/1 -> SlipRatio/1, DriveSpeed/1
  SlipRatio/1 -> CTRL_SlipRatio_na/1
  Divide1/1 -> SlipRatio/2
